simulink model "CURCTL"  (R2022b)
settings: configuration reference "SharedConfig" (kept outside this file)
values from neighbouring files (symbols this model uses):
  DT_CURCTL_C = 0.0001    [CURCTL.sldd]
  FluxLinkage_C = 0.011    [CURCTL.sldd]
  PhaUDAntiWindupGain_C = 25.0    [CURCTL.sldd]
  PhaUDCmdDialEna_C = 0.0    [CURCTL.sldd]
  PhaUDCmdDialVal_C = 0.0    [CURCTL.sldd]
  PhaUDCmdOpenLoop_C = 0.0    [CURCTL.sldd]
  PhaUDGainI_C = 50.0    [CURCTL.sldd]
  PhaUDGainP_C = 0.5    [CURCTL.sldd]
  PhaUMaxVal_C = 12.0    [CURCTL.sldd]
  PhaUQAntiWindupGain_C = 25.0    [CURCTL.sldd]
  PhaUQCmdDialEna_C = 0.0    [CURCTL.sldd]
  PhaUQCmdDialVal_C = 0.0    [CURCTL.sldd]
  PhaUQCmdOpenLoop_C = 2.0    [CURCTL.sldd]
  PhaUQGainI_C = 50.0    [CURCTL.sldd]
  PhaUQGainP_C = 0.5    [CURCTL.sldd]
  StatorInductanceD_C = 0.00018    [CURCTL.sldd]
  StatorInductanceQ_C = 0.00018    [CURCTL.sldd]
undefined symbols (not defined in the file or in its folder): DiscIntNeverNeededParam, DRIVEMODE, slcm
libraries: simulink x3
Description:
  | Generates phase voltage commands to control phase currents
settings Model: DataDictionary=CURCTL.sldd  Creator=Kevin  LastModifiedBy=Max Kolesnikov
settings ConfigSetRef: SourceName=SharedConfig

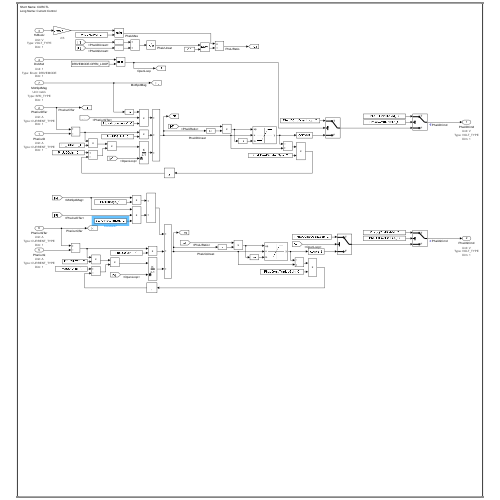
[thumbnail: Simulink's stored preview of the top-level diagram]
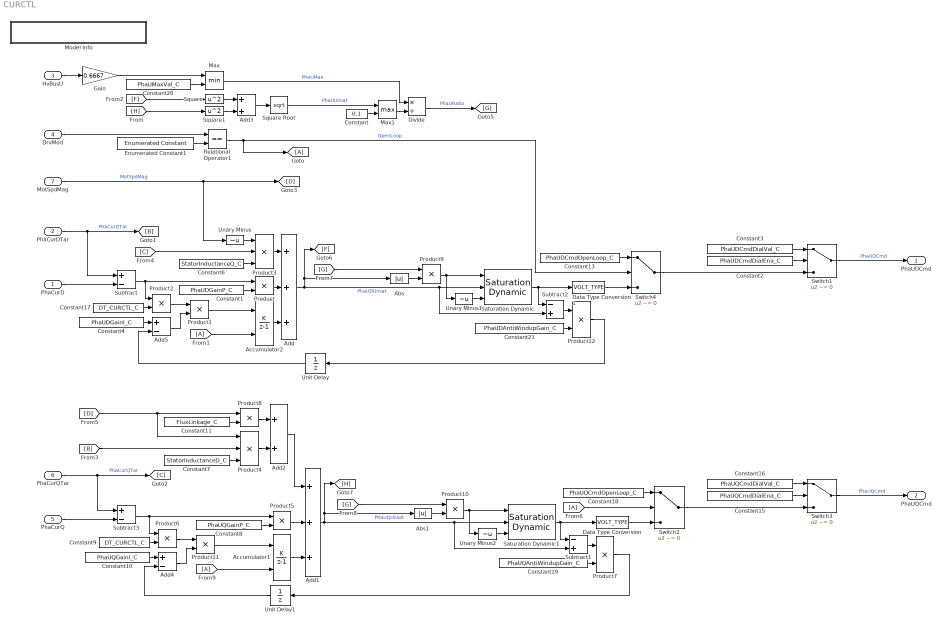
== system CURCTL ==
  PhaCurD : Inport  OutDataTypeStr=CURRENT_TYPE  Unit=A  PortDimensions=1
      settings: AttributesFormatString=|
      | Unit: %<Unit>
      | Type: %<OutDataTypeStr>
      | Dim: %<PortDimensions>
  PhaCurDTar : Inport  Port=2  OutDataTypeStr=CURRENT_TYPE  Unit=A  PortDimensions=1
      settings: AttributesFormatString=|
      | Unit: %<Unit>
      | Type: %<OutDataTypeStr>
      | Dim: %<PortDimensions>
  HvBusU : Inport  Port=3  OutDataTypeStr=VOLT_TYPE  Unit=V  PortDimensions=1
      settings: AttributesFormatString=|
      | Unit: %<Unit>
      | Type: %<OutDataTypeStr>
      | Dim: %<PortDimensions>
  DrvMod : Inport  Port=4  OutDataTypeStr=Enum: DRIVEMODE  Unit=1  PortDimensions=1
      settings: AttributesFormatString=|
      | Unit: %<Unit>
      | Type: %<OutDataTypeStr>
      | Dim: %<PortDimensions>
  PhaCurQ : Inport  Port=5  OutDataTypeStr=CURRENT_TYPE  Unit=A  PortDimensions=1
      settings: AttributesFormatString=|
      | Unit: %<Unit>
      | Type: %<OutDataTypeStr>
      | Dim: %<PortDimensions>
  PhaCurQTar : Inport  Port=6  OutDataTypeStr=CURRENT_TYPE  Unit=A  PortDimensions=1
      settings: AttributesFormatString=|
      | Unit: %<Unit>
      | Type: %<OutDataTypeStr>
      | Dim: %<PortDimensions>
  MotSpdMag : Inport  Port=7  OutDataTypeStr=SPD_TYPE  Unit=rad/s  PortDimensions=1
      settings: AttributesFormatString=|
      | Unit: %<Unit>
      | Type: %<OutDataTypeStr>
      | Dim: %<PortDimensions>
  Abs : Abs  SaturateOnIntegerOverflow=off
  Abs1 : Abs  SaturateOnIntegerOverflow=off
  Accumulator1 : DiscreteIntegrator  IntegratorMethod=Accumulation: Forward Euler  ExternalReset=level  SampleTime=-1  ICPrevOutput=DiscIntNeverNeededParam  ICPrevScaledInput=DiscIntNeverNeededParam
  Accumulator2 : DiscreteIntegrator  IntegratorMethod=Accumulation: Forward Euler  ExternalReset=level  SampleTime=-1  ICPrevOutput=DiscIntNeverNeededParam  ICPrevScaledInput=DiscIntNeverNeededParam
  Add : Sum  Inputs=+++
  Add1 : Sum  Inputs=+++
  Add2 : Sum
  Add3 : Sum
  Add4 : Sum  Inputs=+-
  Add5 : Sum  Inputs=+-
  Constant : Constant  Value=0.1  OutDataTypeStr=single
  Constant1 : Constant  Value=PhaUDGainP_C
  Constant10 : Constant  Value=PhaUQGainI_C
  Constant11 : Constant  Value=FluxLinkage_C
  Constant13 : Constant  Value=PhaUDCmdOpenLoop_C
  Constant15 : Constant  Value=PhaUQCmdDialEna_C
  Constant16 : Constant  Value=PhaUQCmdDialVal_C
  Constant17 : Constant  Value=DT_CURCTL_C
  Constant18 : Constant  Value=PhaUQCmdOpenLoop_C
  Constant19 : Constant  Value=PhaUQAntiWindupGain_C
  Constant2 : Constant  Value=PhaUDCmdDialEna_C
  Constant20 : Constant  Value=PhaUMaxVal_C
  Constant21 : Constant  Value=PhaUDAntiWindupGain_C
  Constant3 : Constant  Value=PhaUDCmdDialVal_C
  Constant4 : Constant  Value=PhaUDGainI_C
  Constant6 : Constant  Value=StatorInductanceQ_C
  Constant7 : Constant  Value=StatorInductanceD_C
  Constant8 : Constant  Value=PhaUQGainP_C
  Constant9 : Constant  Value=DT_CURCTL_C
  Data Type Conversion : DataTypeConversion  OutDataTypeStr=VOLT_TYPE  SaturateOnIntegerOverflow=off  RndMeth=Floor
  Data Type Conversion1 : DataTypeConversion  OutDataTypeStr=VOLT_TYPE  SaturateOnIntegerOverflow=off  RndMeth=Floor
  Divide : Product  Inputs=*/
  Enumerated Constant1 : simulink/Sources/Enumerated Constant  OutDataTypeStr=Enum: DRIVEMODE  Value=DRIVEMODE.OPEN_LOOP  SampleTime=inf
  From1 : From
  From6 : From
  From9 : From
  Gain : Gain  Description=2/3  Gain=0.6667  OutDataTypeStr=VOLT_TYPE
      settings: AttributesFormatString=%<Description>
  Goto : Goto
  Max : MinMax  Inputs=2
  Max1 : MinMax  Function=max  Inputs=2
  Model Info : Subsystem  LoadFcn=slcm LoadBlock;  InitFcn=slcm('UpdateAllCMBlocksInThisModelInit')  mask(CMBlock){Frame=off, DisplayStringWithTags=|, MaskDisplayString=Short Name: CURCTL\nLong Name: Current Control, HorizontalTextAlignment=Left, LeftAlignmentValue=0.02}
      mask DisplayStringWithTags=|
      | Short Name: %<ModelName>
      | Long Name: Current Control
      mask prompts: Frame "Simulink:masks:Frame_MP"; DisplayStringWithTags "Simulink:masks:DisplayStringWithTags_MP"; MaskDisplayString "Simulink:masks:MaskDisplayString_MP"; HorizontalTextAlignment "Simulink:masks:HorizontalTextAlignment_MP"; LeftAlignmentValue "Simulink:masks:LeftAlignmentValue_MP"
      mask help: Simulink:masks:CMBlock_MD
      settings: CopyFcn=slcm CopyBlock;  DeleteFcn=slcm Cancel;  PostSaveFcn=slcm('UpdateAllCMBlocksInThisModel')  NameChangeFcn=slcm Rename;  OpenFcn=slcm
      mask Display: text(slResolve(LeftAlignmentValue, gcbh), 0.5, MaskDisplayString, 'HorizontalAlignment', HorizontalTextAlignment)
  Product{,1..2,5..12} (11 alike) : Product
  Product3 : Product  Inputs=***
  Product4 : Product  Inputs=***
  Relational Operator1 : RelationalOperator  Operator===  OutDataTypeStr=boolean  RndMeth=Simplest  InputSameDT=off
  Saturation Dynamic : simulink/Discontinuities/Saturation Dynamic  OutMin=[]  OutMax=[]  OutDataTypeStr=Inherit: Same as second input  OutDataType=fixdt(1, 16)  OutScaling=2^-10  DoSatur=off
  Saturation Dynamic1 : simulink/Discontinuities/Saturation Dynamic  OutMin=[]  OutMax=[]  OutDataTypeStr=Inherit: Same as second input  OutDataType=fixdt(1, 16)  OutScaling=2^-10  DoSatur=off
  Square : Math  Operator=square
  Square Root : Sqrt
  Square1 : Math  Operator=square
  Subtract : Sum  Inputs=+-
  Subtract1 : Sum  Inputs=-+
  Subtract2 : Sum  Inputs=-+
  Subtract3 : Sum  Inputs=+-
  Switch{1..4} (4 alike) : Switch  Criteria=u2 ~= 0  SaturateOnIntegerOverflow=off  InputSameDT=off
  Unary Minus : UnaryMinus
  Unary Minus1 : UnaryMinus
  Unary Minus2 : UnaryMinus
  Unit Delay : UnitDelay  SampleTime=-1  HasFrameUpgradeWarning=on
  Unit Delay1 : UnitDelay  SampleTime=-1  HasFrameUpgradeWarning=on
  PhaUDCmd : Outport  OutDataTypeStr=VOLT_TYPE  Unit=V  PortDimensions=1
      settings: AttributesFormatString=|
      | Unit: %<Unit>
      | Type: %<OutDataTypeStr>
      | Dim: %<PortDimensions>
  PhaUQCmd : Outport  Port=2  OutDataTypeStr=VOLT_TYPE  Unit=V  PortDimensions=1
      settings: AttributesFormatString=|
      | Unit: %<Unit>
      | Type: %<OutDataTypeStr>
      | Dim: %<PortDimensions>
  wires:
  PhaCurD/1 -> Subtract/2
  Switch1/1 -> PhaUDCmd/1  "PhaUDCmd"
  Constant2/1 -> Switch1/2
  Constant3/1 -> Switch1/1
  PhaCurDTar/1 -> [B], Subtract/1  "PhaCurDTar"
  HvBusU/1 -> Gain/1
  Subtract/1 -> Product2/1, Product/1
  Constant1/1 -> Product/2
  DrvMod/1 -> Relational Operator1/1
  Product/1 -> Add/2
  Product5/1 -> Add1/2
  Constant9/1 -> Product6/2
  Relational Operator1/1 -> Switch4/2, Goto/1  "OpenLoop"
  Constant8/1 -> Product5/2
  Switch4/1 -> Switch1/3
  PhaCurQTar/1 -> [C], Subtract3/1  "PhaCurQTar"
  PhaCurQ/1 -> Subtract3/2
  Switch2/1 -> Switch3/3
  Constant16/1 -> Switch3/1
  Constant15/1 -> Switch3/2
  Switch3/1 -> PhaUQCmd/1  "PhaUQCmd"
  Subtract3/1 -> Product5/1, Product6/1
  Product3/1 -> Add/1
  Unary Minus/1 -> Product3/1
  MotSpdMag/1 -> [D], Unary Minus/1  "MotSpdMag"
  Constant6/1 -> Product3/3
  Constant7/1 -> Product4/3
  Constant11/1 -> Product8/2
  Product8/1 -> Add2/1
  Product4/1 -> Add2/2
  Add2/1 -> Add1/1
  [B] -> Product4/2
  [C] -> Product3/2
  [D] -> Product4/1, Product8/1
  Constant13/1 -> Switch4/1
  Constant18/1 -> Switch2/1
  Enumerated Constant1/1 -> Relational Operator1/2
  Max/1 -> Divide/1  "PhaUMax"
  Data Type Conversion1/1 -> Switch4/3
  From9/1 -> Accumulator1/2
  Gain/1 -> Max/1
  Constant20/1 -> Max/2
  Data Type Conversion/1 -> Switch2/3
  Saturation Dynamic/1 -> Subtract2/1, Data Type Conversion1/1
  Unary Minus1/1 -> Saturation Dynamic/3
  Saturation Dynamic1/1 -> Subtract1/1, Data Type Conversion/1
  Add/1 -> [F], Abs/1, Subtract2/2, Saturation Dynamic/2  "PhaUDUnsat"
  Add1/1 -> Saturation Dynamic1/2, Subtract1/2, Abs1/1, [H]  "PhaUQUnsat"
  [F] -> Square/1
  [H] -> Square1/1
  Square/1 -> Add3/1
  Square1/1 -> Add3/2
  Add3/1 -> Square Root/1
  Square Root/1 -> Max1/1  "PhaUUnsat"
  Max1/1 -> Divide/2
  Constant/1 -> Max1/2
  Divide/1 -> [G]  "PhaURatio"
  [G] -> Product9/1
  Abs/1 -> Product9/2
  Product9/1 -> Saturation Dynamic/1, Unary Minus1/1
  Product10/1 -> Saturation Dynamic1/1, Unary Minus2/1
  Abs1/1 -> Product10/2
  [G] -> Product10/1
  Unary Minus2/1 -> Saturation Dynamic1/3
  Accumulator1/1 -> Add1/3
  Product7/1 -> Unit Delay1/1
  Constant10/1 -> Add4/1
  Unit Delay1/1 -> Add4/2
  Subtract1/1 -> Product7/1
  Product6/1 -> Product11/1
  Add4/1 -> Product11/2
  Product11/1 -> Accumulator1/1
  Constant19/1 -> Product7/2
  Constant21/1 -> Product12/2
  Subtract2/1 -> Product12/1
  Product12/1 -> Unit Delay/1
  Product1/1 -> Accumulator2/1
  Add5/1 -> Product1/2
  Product2/1 -> Product1/1
  Unit Delay/1 -> Add5/2
  Constant4/1 -> Add5/1
  Accumulator2/1 -> Add/3
  From1/1 -> Accumulator2/2
  Constant17/1 -> Product2/2
  From6/1 -> Switch2/2

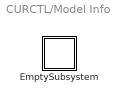
== system CURCTL/Model Info ==
  EmptySubsystem : Subsystem

== system CURCTL/Model Info/EmptySubsystem ==
